simulink library "aausat3_lib"  (Simulink 8.3)
settings: Solver=ode45  StartTime=0.0  StopTime=10.0  RelTol=1e-3
undefined symbols (not defined in the file or in its folder): A_wire_mt, albedo_wrapper, alpha_0_mt, bias_gyro, bias_mag, bias_sun, Cd, coil_dim, Dim, f_sample, G, heading_gyro, heading_mag, M_earth, M_moon, M_sun, magnitude, n_mt, noise_gyro, noise_mag, noise_sun, nr_sample_sun, otoquest, otoquest_with_pro, q_method, qmethod, redfac, refldata, s_freq_gyro, s_freq_mag, s_freq_sun, sigma_0_mt, solar_absorb_coeff, solar_m_flux, SVD_method, T_0_mt, theta_e, tilt_gyro, tilt_mag, Ts
undefined symbols (not defined in the file): Actuator_Duty_Cycle_coil, Actuator_Frequency_coil, Dimensions_coil, mean_refl, Number_of_Windings_coil, rho, sim_par, svd_weigth, Wire_Cross_Sectional_Area_coil, Wire_Resistivity_Base_Temperature_coil, Wire_Resistivity_coil, Wire_Resistivity_Temperature_Coefficient_coil
libraries: aausat3_lib x118, simulink_extras x3
(part 4 of 4)

== system aausat3_lib/On-board Software/Orbit and Magnetic field models/initial time ==
  Initial time in (JD) : Inport
  TLE : Inport  Port=2
  Demux : Demux  Outputs=12
  Mux1 : Mux  Inputs=12
  Switch : Switch  Criteria=u2 > Threshold
  "TLE -> JD converter SW" : aausat3_lib/Other Model Utilities/TLE -> JD converter  SystemSampleTime=-1
  Terminator : Terminator
  Initial time out (JD) : Outport
  wires:
  Mux1/1 -> Terminator/1
  Switch/1 -> Initial time out (JD)/1
  Initial time in (JD)/1 -> Switch/1, Switch/2
  TLE/1 -> Demux/1
  Demux/2 -> Mux1/2
  Demux/3 -> Mux1/3
  Demux/4 -> Mux1/4
  Demux/5 -> Mux1/5
  Demux/6 -> Mux1/6
  Demux/7 -> Mux1/7
  Demux/8 -> Mux1/8
  Demux/9 -> Mux1/9
  Demux/10 -> Mux1/10
  Demux/11 -> Mux1/11
  Demux/12 -> Mux1/12
  Demux/1 -> "TLE -> JD converter SW"/1
  "TLE -> JD converter SW"/1 -> Switch/3, Mux1/1

== system aausat3_lib/Orbit and Ephemeris/(IGRF) Magnetic field/Magnetic field model ==
  R_sc(E) : Inport
  S-Function : S-Function  FunctionName=igrfS  Parameters=2009,13  EnableBusSupport=off
  B(E) : Outport
  wires:
  R_sc(E)/1 -> S-Function/1
  S-Function/1 -> B(E)/1

== system aausat3_lib/Orbit and Ephemeris/Albedo/Earth Albedo Model ==
  r_sat_ecef : Inport  SampleTime=Ts
  r_sun_ecef : Inport  Port=2  SampleTime=Ts
  AlbedoFcn : MATLABFcn  MATLABFcn=albedo_wrapper(u(1:3),u(4:6),refldata,redfac)  OutputDimensions=[sy sx]  OutputSignalType=real  Output1D=off
  Mux : Mux  Inputs=2
  Zero-Order Hold1 : ZeroOrderHold  SampleTime=Ts
  Zero-Order Hold2 : ZeroOrderHold  SampleTime=Ts
  a : Outport
  wires:
  r_sat_ecef/1 -> Zero-Order Hold2/1
  AlbedoFcn/1 -> a/1
  r_sun_ecef/1 -> Zero-Order Hold1/1
  Zero-Order Hold2/1 -> Mux/1
  Zero-Order Hold1/1 -> Mux/2
  Mux/1 -> AlbedoFcn/1

== system aausat3_lib/Orbit and Ephemeris/Ephemeris/Moon Position ==
  t(JD)1 : Inport
  MATLAB Function : MATLAB Function  TreatAsAtomicUnit=on
  R_m(I) : Outport
  wires:
  MATLAB Function/1(y) -> R_m(I)/1
  t(JD)1/1 -> MATLAB Function/1(u)

== system aausat3_lib/Orbit and Ephemeris/Ephemeris/Sun Position ==
  t(JD) : Inport
  MATLAB Function : MATLAB Function  TreatAsAtomicUnit=on
  R_s(I) : Outport
  wires:
  MATLAB Function/1(y) -> R_s(I)/1
  t(JD)/1 -> MATLAB Function/1(u)

== system aausat3_lib/Orbit and Ephemeris/Orbit and Magnetic field models/initial time ==
  Initial time in (JD) : Inport
  TLE : Inport  Port=2
  Demux : Demux  Outputs=12
  Mux1 : Mux  Inputs=12
  Switch : Switch  Criteria=u2 > Threshold
  "TLE -> JD converter" : aausat3_lib/Other Model Utilities/TLE -> JD converter
  Terminator : Terminator
  Initial time out (JD) : Outport
  wires:
  "TLE -> JD converter"/1 -> Mux1/1, Switch/3
  Demux/1 -> "TLE -> JD converter"/1
  Demux/12 -> Mux1/12
  Demux/11 -> Mux1/11
  Demux/10 -> Mux1/10
  Demux/9 -> Mux1/9
  Demux/8 -> Mux1/8
  Demux/7 -> Mux1/7
  Demux/6 -> Mux1/6
  Demux/5 -> Mux1/5
  Demux/4 -> Mux1/4
  Demux/3 -> Mux1/3
  Demux/2 -> Mux1/2
  TLE/1 -> Demux/1
  Initial time in (JD)/1 -> Switch/2, Switch/1
  Switch/1 -> Initial time out (JD)/1
  Mux1/1 -> Terminator/1

== system aausat3_lib/Other Model Utilities/Exposed area/Projection Matrix1 ==
  n-vector : Inport
  Add : Sum  Inputs=+++
  Demux : Demux  Outputs=3
  Gain{1..6} (6 alike) : Gain  Gain=-1
  Math Funcion : Math  Operator=square  SaturateOnIntegerOverflow=on
  Math Function : Math  Operator=reciprocal  SaturateOnIntegerOverflow=on
  Math Function1 : Math  Operator=square  SaturateOnIntegerOverflow=on
  Math Function2 : Math  Operator=square  SaturateOnIntegerOverflow=on
  Mux : Mux  Inputs=9
  Product1 : Product  RndMeth=Zero
  Product2 : Product  RndMeth=Zero
  Product3 : Product  RndMeth=Zero
  Prouct : Product  RndMeth=Zero
  Reshape : Reshape  OutputDimensionality=Customize  OutputDimensions=[3,3]
  Sum : Sum  Inputs=|++
  Sum1 : Sum  Inputs=+|+
  Sum2 : Sum  Inputs=++|
  P matrix : Outport
  wires:
  Prouct/1 -> P matrix/1
  Reshape/1 -> Prouct/2
  Add/1 -> Math Function/1
  Math Function/1 -> Prouct/1
  n-vector/1 -> Demux/1
  Mux/1 -> Reshape/1
  Math Function1/1 -> Add/2, Sum/1, Sum2/2
  Math Function2/1 -> Add/3, Sum/2, Sum1/2
  Math Funcion/1 -> Add/1, Sum2/1, Sum1/1
  Sum1/1 -> Mux/5
  Sum2/1 -> Mux/9
  Sum/1 -> Mux/1
  Product3/1 -> Gain6/1, Gain4/1
  Product2/1 -> Gain5/1, Gain2/1
  Product1/1 -> Gain3/1, Gain1/1
  Gain6/1 -> Mux/8
  Gain5/1 -> Mux/7
  Gain4/1 -> Mux/6
  Gain3/1 -> Mux/4
  Gain2/1 -> Mux/3
  Gain1/1 -> Mux/2
  Demux/3 -> Product3/2, Math Function2/1, Product2/2
  Demux/2 -> Product3/1, Product1/2, Math Function1/1
  Demux/1 -> Product2/1, Product1/1, Math Funcion/1

== system aausat3_lib/Other Model Utilities/Geocentric to  Geodetic Latitude/alt ==
  l_point : Inport
  delta_lambda : Inport  Port=2
  Product : Product  RndMeth=Zero
  Trigonometric Function1 : Trigonometry  Operator=cos
  alt : Outport
  wires:
  Trigonometric Function1/1 -> Product/2
  l_point/1 -> Product/1
  Product/1 -> alt/1
  delta_lambda/1 -> Trigonometric Function1/1

== system aausat3_lib/Other Model Utilities/Geocentric to  Geodetic Latitude/delt_mu ==
  l_point : Inport
  alt : Inport  Port=2
  delta_lambda : Inport  Port=3
  rho_alpha : Inport  Port=4
  Product : Product  RndMeth=Zero
  Sum1 : Sum  Inputs=|++
  Trigonometric Function1 : Trigonometry  Operator=atan2
  Trigonometric Function2 : Trigonometry
  delt_mu : Outport
  wires:
  Product/1 -> Trigonometric Function1/1
  l_point/1 -> Product/1
  delta_lambda/1 -> Trigonometric Function2/1
  alt/1 -> Sum1/1
  Sum1/1 -> Trigonometric Function1/2
  rho_alpha/1 -> Sum1/2
  Trigonometric Function1/1 -> delt_mu/1
  Trigonometric Function2/1 -> Product/2

== system aausat3_lib/Other Model Utilities/Geocentric to  Geodetic Latitude/delta_lambda ==
  mu_alpha : Inport
  lambda : Inport  Port=2
  Sum1 : Sum  Inputs=|+-
  delta_lambda : Outport
  wires:
  lambda/1 -> Sum1/2
  mu_alpha/1 -> Sum1/1
  Sum1/1 -> delta_lambda/1

== system aausat3_lib/Other Model Utilities/Geocentric to  Geodetic Latitude/denom ==
  mu_alpha : Inport
  eps : Inport  Port=2
  Constant : Constant
  Math Function : Math  Operator=sqrt  SaturateOnIntegerOverflow=on
  Product1 : Product  Inputs=4  RndMeth=Zero
  Sum1 : Sum  Inputs=|+-
  Trigonometric Function1 : Trigonometry
  denom : Outport
  wires:
  Math Function/1 -> denom/1
  Sum1/1 -> Math Function/1
  Constant/1 -> Sum1/1
  Product1/1 -> Sum1/2
  eps/1 -> Product1/2, Product1/1
  Trigonometric Function1/1 -> Product1/4, Product1/3
  mu_alpha/1 -> Trigonometric Function1/1

== system aausat3_lib/Other Model Utilities/Geocentric to  Geodetic Latitude/e ==
  Constant : Constant  Value=F
  Sum : Sum  Inputs=-+
  f : Constant
  e : Outport
  wires:
  Sum/1 -> e/1
  Constant/1 -> Sum/1
  f/1 -> Sum/2

== system aausat3_lib/Other Model Utilities/Geocentric to  Geodetic Latitude/e^4 ==
  e : Inport
  Constant : Constant
  Math Function : Math  Operator=sqrt  SaturateOnIntegerOverflow=on
  Product1 : Product  RndMeth=Zero
  Sum1 : Sum  Inputs=|+-
  eps : Outport
  wires:
  e/1 -> Product1/1, Product1/2
  Product1/1 -> Sum1/2
  Constant/1 -> Sum1/1
  Sum1/1 -> Math Function/1
  Math Function/1 -> eps/1

== system aausat3_lib/Other Model Utilities/Geocentric to  Geodetic Latitude/l_point ==
  dist to body : Inport
  r_alpha : Inport  Port=2
  Sum1 : Sum  Inputs=|+-
  l_point : Outport
  wires:
  Sum1/1 -> l_point/1
  dist to body/1 -> Sum1/1
  r_alpha/1 -> Sum1/2

== system aausat3_lib/Other Model Utilities/Geocentric to  Geodetic Latitude/mu_alpha ==
  R^2 : Inport
  x_alpha : Inport  Port=2
  e : Inport  Port=3
  lambda : Inport  Port=4
  Math Function1 : Math  Operator=sqrt  SaturateOnIntegerOverflow=on
  Product1 : Product  RndMeth=Zero
  Product2 : Product  RndMeth=Zero
  Product3 : Product  RndMeth=Zero
  Sign : Signum
  Sum1 : Sum  Inputs=+-|
  Trigonometric Function1 : Trigonometry  Operator=atan2
  mu_alpha : Outport
  wires:
  x_alpha/1 -> Product3/1, Product2/1, Product2/2  "x_alpha"
  Product2/1 -> Sum1/2
  Sum1/1 -> Math Function1/1
  Math Function1/1 -> Trigonometric Function1/1
  Product3/1 -> Trigonometric Function1/2
  e/1 -> Product3/2
  R^2/1 -> Sum1/1
  Product1/1 -> mu_alpha/1  "mu_alpha"
  lambda/1 -> Sign/1
  Trigonometric Function1/1 -> Product1/1  "mu_alpha"
  Sign/1 -> Product1/2

== system aausat3_lib/Other Model Utilities/Geocentric to  Geodetic Latitude/r_alpha ==
  lambda : Inport
  x_alpha : Inport  Port=2
  Product : Product  Inputs=*/  RndMeth=Zero
  Trigonometric Function1 : Trigonometry  Operator=cos
  r_alpha : Outport
  wires:
  Trigonometric Function1/1 -> Product/2
  lambda/1 -> Trigonometric Function1/1
  x_alpha/1 -> Product/1
  Product/1 -> r_alpha/1

== system aausat3_lib/Other Model Utilities/Geocentric to  Geodetic Latitude/rho_alpha ==
  R : Inport
  denom : Inport  Port=2
  eps : Inport  Port=3
  Constant1 : Constant
  Product1 : Product  Inputs=**/  RndMeth=Zero
  Product2 : Product  Inputs=**  RndMeth=Zero
  Product3 : Product  Inputs=3  RndMeth=Zero
  Sum1 : Sum  Inputs=|+-
  rho_alpha : Outport
  wires:
  denom/1 -> Product3/1, Product3/2, Product3/3
  Constant1/1 -> Sum1/1
  Sum1/1 -> Product1/2
  R/1 -> Product1/1
  eps/1 -> Product2/1, Product2/2
  Product1/1 -> rho_alpha/1
  Product2/1 -> Sum1/2
  Product3/1 -> Product1/3

== system aausat3_lib/Other Model Utilities/Geocentric to  Geodetic Latitude/square e ==
  e : Inport
  Product1 : Product  Inputs=**  RndMeth=Zero
  e^2 : Outport
  wires:
  Product1/1 -> e^2/1
  e/1 -> Product1/2, Product1/1

== system aausat3_lib/Other Model Utilities/Geocentric to  Geodetic Latitude/square e1 ==
  R : Inport
  Product1 : Product  Inputs=**  RndMeth=Zero
  R^2 : Outport
  wires:
  R/1 -> Product1/1, Product1/2
  Product1/1 -> R^2/1

== system aausat3_lib/Other Model Utilities/Geocentric to  Geodetic Latitude/x_alpha ==
  R : Inport
  t_lat : Inport  Port=2
  e : Inport  Port=3
  e^2 : Inport  Port=4
  Math Function : Math  Operator=sqrt  SaturateOnIntegerOverflow=on
  Product : Product  RndMeth=Zero
  Product1 : Product  Inputs=*/*  RndMeth=Zero
  Sum : Sum  Inputs=|++
  x_alpha : Outport
  wires:
  t_lat/1 -> Product/1, Product/2  "t_lat"
  Product/1 -> Sum/1
  Sum/1 -> Math Function/1
  Math Function/1 -> Product1/2
  R/1 -> Product1/1
  e/1 -> Product1/3
  Product1/1 -> x_alpha/1  "x_alpha"
  e^2/1 -> Sum/2

== system aausat3_lib/Other Model Utilities/Geodetic to  Geocentric Latitude/Radius at Geocentric Latitude ==
  lambda_s : Inport
  Constant : Constant
  Math Function : Math  Operator=sqrt  SaturateOnIntegerOverflow=on
  Product1 : Product  Inputs=*/  RndMeth=Zero
  Product2 : Product  Inputs=3  RndMeth=Zero
  Product3 : Product  Inputs=**/  RndMeth=Zero
  Product4 : Product  RndMeth=Zero
  Re : Constant  Value=R
  Sum : Sum  Inputs=+-
  Sum1 : Sum  Inputs=-+|
  Sum2 : Sum  Inputs=++|
  Trigonometric Function : Trigonometry
  deg->rad : Gain  Gain=pi/180
  f : Constant  Value=F
  r_s : Outport
  wires:
  Product4/1 -> Product1/2
  lambda_s/1 -> deg->rad/1
  Constant/1 -> Product1/1, Sum/1, Sum1/1, Sum2/1
  f/1 -> Sum/2
  Sum/1 -> Product4/1, Product4/2
  Product1/1 -> Sum1/2
  Sum1/1 -> Product2/3
  Trigonometric Function/1 -> Product2/1, Product2/2
  Product2/1 -> Sum2/2
  Sum2/1 -> Product3/3
  Re/1 -> Product3/2, Product3/1
  Product3/1 -> Math Function/1
  Math Function/1 -> r_s/1
  deg->rad/1 -> Trigonometric Function/1

== system aausat3_lib/Other Model Utilities/Store data/enable ==
  In : Inport
  Constant : Constant  Value=enable_signal
  Ground : Ground
  Switch : Switch  Threshold=1
  Out : Outport
  wires:
  Constant/1 -> Switch/2
  Ground/1 -> Switch/3
  In/1 -> Switch/1
  Switch/1 -> Out/1

== system aausat3_lib/Other Model Utilities/Store data/enable1 ==
  In : Inport
  Constant : Constant  Value=enable_signal
  Ground : Ground
  Switch : Switch  Threshold=1
  Out : Outport
  wires:
  Constant/1 -> Switch/2
  Ground/1 -> Switch/3
  In/1 -> Switch/1
  Switch/1 -> Out/1

== system aausat3_lib/Other Model Utilities/Store data/enable10 ==
  In : Inport
  Constant : Constant  Value=enable_signal
  Ground : Ground
  Switch : Switch  Threshold=1
  Out : Outport
  wires:
  Constant/1 -> Switch/2
  Ground/1 -> Switch/3
  In/1 -> Switch/1
  Switch/1 -> Out/1

== system aausat3_lib/Other Model Utilities/Store data/enable11 ==
  In : Inport
  Constant : Constant  Value=enable_signal
  Ground : Ground
  Switch : Switch  Threshold=1
  Out : Outport
  wires:
  Constant/1 -> Switch/2
  Ground/1 -> Switch/3
  In/1 -> Switch/1
  Switch/1 -> Out/1

== system aausat3_lib/Other Model Utilities/Store data/enable12 ==
  In : Inport
  Constant : Constant  Value=enable_signal
  Ground : Ground
  Switch : Switch  Threshold=1
  Out : Outport
  wires:
  Constant/1 -> Switch/2
  Ground/1 -> Switch/3
  In/1 -> Switch/1
  Switch/1 -> Out/1

== system aausat3_lib/Other Model Utilities/Store data/enable13 ==
  In : Inport
  Constant : Constant  Value=enable_signal
  Ground : Ground
  Switch : Switch  Threshold=1
  Out : Outport
  wires:
  Constant/1 -> Switch/2
  Ground/1 -> Switch/3
  In/1 -> Switch/1
  Switch/1 -> Out/1

== system aausat3_lib/Other Model Utilities/Store data/enable14 ==
  In : Inport
  Constant : Constant  Value=enable_signal
  Ground : Ground
  Switch : Switch  Threshold=1
  Out : Outport
  wires:
  Constant/1 -> Switch/2
  Ground/1 -> Switch/3
  In/1 -> Switch/1
  Switch/1 -> Out/1

== system aausat3_lib/Other Model Utilities/Store data/enable15 ==
  In : Inport
  Constant : Constant  Value=enable_signal
  Ground : Ground
  Switch : Switch  Threshold=1
  Out : Outport
  wires:
  Constant/1 -> Switch/2
  Ground/1 -> Switch/3
  In/1 -> Switch/1
  Switch/1 -> Out/1

== system aausat3_lib/Other Model Utilities/Store data/enable16 ==
  In : Inport
  Constant : Constant  Value=enable_signal
  Ground : Ground
  Switch : Switch  Threshold=1
  Out : Outport
  wires:
  Constant/1 -> Switch/2
  Ground/1 -> Switch/3
  In/1 -> Switch/1
  Switch/1 -> Out/1

== system aausat3_lib/Other Model Utilities/Store data/enable17 ==
  In : Inport
  Constant : Constant  Value=enable_signal
  Ground : Ground
  Switch : Switch  Threshold=1
  Out : Outport
  wires:
  Constant/1 -> Switch/2
  Ground/1 -> Switch/3
  In/1 -> Switch/1
  Switch/1 -> Out/1

== system aausat3_lib/Other Model Utilities/Store data/enable18 ==
  In : Inport
  Constant : Constant  Value=enable_signal
  Ground : Ground
  Switch : Switch  Threshold=1
  Out : Outport
  wires:
  Constant/1 -> Switch/2
  Ground/1 -> Switch/3
  In/1 -> Switch/1
  Switch/1 -> Out/1

== system aausat3_lib/Other Model Utilities/Store data/enable19 ==
  In : Inport
  Constant : Constant  Value=enable_signal
  Ground : Ground
  Switch : Switch  Threshold=1
  Out : Outport
  wires:
  Constant/1 -> Switch/2
  Ground/1 -> Switch/3
  In/1 -> Switch/1
  Switch/1 -> Out/1

== system aausat3_lib/Other Model Utilities/Store data/enable2 ==
  In : Inport
  Constant : Constant  Value=enable_signal
  Ground : Ground
  Switch : Switch  Threshold=1
  Out : Outport
  wires:
  Constant/1 -> Switch/2
  Ground/1 -> Switch/3
  In/1 -> Switch/1
  Switch/1 -> Out/1

== system aausat3_lib/Other Model Utilities/Store data/enable21 ==
  In : Inport
  Constant : Constant  Value=enable_signal
  Ground : Ground
  Switch : Switch  Threshold=1
  Out : Outport
  wires:
  Constant/1 -> Switch/2
  Ground/1 -> Switch/3
  In/1 -> Switch/1
  Switch/1 -> Out/1

== system aausat3_lib/Other Model Utilities/Store data/enable22 ==
  In : Inport
  Constant : Constant  Value=enable_signal
  Ground : Ground
  Switch : Switch  Threshold=1
  Out : Outport
  wires:
  Constant/1 -> Switch/2
  Ground/1 -> Switch/3
  In/1 -> Switch/1
  Switch/1 -> Out/1

== system aausat3_lib/Other Model Utilities/Store data/enable23 ==
  In : Inport
  Constant : Constant  Value=enable_signal
  Ground : Ground
  Switch : Switch  Threshold=1
  Out : Outport
  wires:
  Constant/1 -> Switch/2
  Ground/1 -> Switch/3
  In/1 -> Switch/1
  Switch/1 -> Out/1

== system aausat3_lib/Other Model Utilities/Store data/enable24 ==
  In : Inport
  Constant : Constant  Value=enable_signal
  Ground : Ground
  Switch : Switch  Threshold=1
  Out : Outport
  wires:
  Constant/1 -> Switch/2
  Ground/1 -> Switch/3
  In/1 -> Switch/1
  Switch/1 -> Out/1

== system aausat3_lib/Other Model Utilities/Store data/enable25 ==
  In : Inport
  Constant : Constant  Value=enable_signal
  Ground : Ground
  Switch : Switch  Threshold=1
  Out : Outport
  wires:
  Constant/1 -> Switch/2
  Ground/1 -> Switch/3
  In/1 -> Switch/1
  Switch/1 -> Out/1

== system aausat3_lib/Other Model Utilities/Store data/enable26 ==
  In : Inport
  Constant : Constant  Value=enable_signal
  Ground : Ground
  Switch : Switch  Threshold=1
  Out : Outport
  wires:
  Constant/1 -> Switch/2
  Ground/1 -> Switch/3
  In/1 -> Switch/1
  Switch/1 -> Out/1

== system aausat3_lib/Other Model Utilities/Store data/enable27 ==
  In : Inport
  Constant : Constant  Value=enable_signal
  Ground : Ground
  Switch : Switch  Threshold=1
  Out : Outport
  wires:
  Constant/1 -> Switch/2
  Ground/1 -> Switch/3
  In/1 -> Switch/1
  Switch/1 -> Out/1

== system aausat3_lib/Other Model Utilities/Store data/enable28 ==
  In : Inport
  Constant : Constant  Value=enable_signal
  Ground : Ground
  Switch : Switch  Threshold=1
  Out : Outport
  wires:
  Constant/1 -> Switch/2
  Ground/1 -> Switch/3
  In/1 -> Switch/1
  Switch/1 -> Out/1

== system aausat3_lib/Other Model Utilities/Store data/enable29 ==
  In : Inport
  Constant : Constant  Value=enable_signal
  Ground : Ground
  Switch : Switch  Threshold=1
  Out : Outport
  wires:
  Constant/1 -> Switch/2
  Ground/1 -> Switch/3
  In/1 -> Switch/1
  Switch/1 -> Out/1

== system aausat3_lib/Other Model Utilities/Store data/enable3 ==
  In : Inport
  Constant : Constant  Value=enable_signal
  Ground : Ground
  Switch : Switch  Threshold=1
  Out : Outport
  wires:
  Constant/1 -> Switch/2
  Ground/1 -> Switch/3
  In/1 -> Switch/1
  Switch/1 -> Out/1

== system aausat3_lib/Other Model Utilities/Store data/enable4 ==
  In : Inport
  Constant : Constant  Value=enable_signal
  Ground : Ground
  Switch : Switch  Threshold=1
  Out : Outport
  wires:
  Constant/1 -> Switch/2
  Ground/1 -> Switch/3
  In/1 -> Switch/1
  Switch/1 -> Out/1

== system aausat3_lib/Other Model Utilities/Store data/enable5 ==
  In : Inport
  Constant : Constant  Value=enable_signal
  Ground : Ground
  Switch : Switch  Threshold=1
  Out : Outport
  wires:
  Constant/1 -> Switch/2
  Ground/1 -> Switch/3
  In/1 -> Switch/1
  Switch/1 -> Out/1

== system aausat3_lib/Other Model Utilities/Store data/enable6 ==
  In : Inport
  Constant : Constant  Value=enable_signal
  Ground : Ground
  Switch : Switch  Threshold=1
  Out : Outport
  wires:
  Constant/1 -> Switch/2
  Ground/1 -> Switch/3
  In/1 -> Switch/1
  Switch/1 -> Out/1

== system aausat3_lib/Other Model Utilities/Store data/enable7 ==
  In : Inport
  Constant : Constant  Value=enable_signal
  Ground : Ground
  Switch : Switch  Threshold=1
  Out : Outport
  wires:
  Constant/1 -> Switch/2
  Ground/1 -> Switch/3
  In/1 -> Switch/1
  Switch/1 -> Out/1

== system aausat3_lib/Other Model Utilities/Store data/enable8 ==
  In : Inport
  Constant : Constant  Value=enable_signal
  Ground : Ground
  Switch : Switch  Threshold=1
  Out : Outport
  wires:
  Constant/1 -> Switch/2
  Ground/1 -> Switch/3
  In/1 -> Switch/1
  Switch/1 -> Out/1

== system aausat3_lib/Other Model Utilities/Store data/enable9 ==
  In : Inport
  Constant : Constant  Value=enable_signal
  Ground : Ground
  Switch : Switch  Threshold=1
  Out : Outport
  wires:
  Constant/1 -> Switch/2
  Ground/1 -> Switch/3
  In/1 -> Switch/1
  Switch/1 -> Out/1

== system aausat3_lib/Sensor Emulation/Magnetometers/Vector rotation by q ==
  q : Inport
  V : Inport  Port=2
  Constant : Constant  Value=0
  Demux : Demux  Outputs=3
  Demux1 : Demux
  Mux : Mux
  Mux1 : Mux  Inputs=3
  Quaternion inverter : Subsystem
  Quaternion mulitiplication : S-Function  FunctionName=qmul  EnableBusSupport=off
  Quaternion mulitiplication1 : S-Function  FunctionName=qmul  EnableBusSupport=off
  Terminator : Terminator
  q'Vq : Outport
  wires:
  Mux1/1 -> q'Vq/1
  Demux1/4 -> Terminator/1
  Demux1/3 -> Mux1/3
  Demux1/2 -> Mux1/2
  Demux1/1 -> Mux1/1
  Quaternion mulitiplication1/1 -> Demux1/1
  Quaternion mulitiplication/1 -> Quaternion mulitiplication1/1
  Mux/1 -> Quaternion mulitiplication/2
  Constant/1 -> Mux/4
  Demux/3 -> Mux/3
  Demux/2 -> Mux/2
  Demux/1 -> Mux/1
  V/1 -> Demux/1
  Quaternion inverter/1(q^-1) -> Quaternion mulitiplication/1
  q/1 -> Quaternion mulitiplication1/2, Quaternion inverter/1(q)

== system aausat3_lib/Sensor Emulation/Sun sensors/Cartesian to Spherical ==
  x : Inport  PortDimensions=1
  y : Inport  Port=2  PortDimensions=1
  z : Inport  Port=3  PortDimensions=1
  Mux : Mux  Inputs=2
  Mux1 : Mux  Inputs=2
  calc phi : Fcn  Expr=atan2(u[1],u[2])
  calc r : Fcn  Expr=hypot(u[1],u[2])
  calc theta : Fcn  Expr=atan2(u[2],u[1])
  temp : Fcn  Expr=hypot(u[1],u[2])
  "r " : Outport  InitialOutput=0
  theta : Outport  Port=2  InitialOutput=0
  phi : Outport  Port=3  InitialOutput=0
  wires:
  calc theta/1 -> theta/1
  calc phi/1 -> phi/1
  y/1 -> Mux/2
  x/1 -> Mux/1
  temp/1 -> Mux1/1
  z/1 -> Mux1/2
  calc r/1 -> "r "/1
  Mux/1 -> calc theta/1, temp/1
  Mux1/1 -> calc phi/1, calc r/1

== system aausat3_lib/Sensor Emulation/Sun sensors/Spherical to Cartesian ==
  r : Inport  PortDimensions=1
  theta : Inport  Port=2  PortDimensions=1
  phi : Inport  Port=3  PortDimensions=1
  Mux : Mux  Inputs=2
  Mux1 : Mux  Inputs=2
  temp : Fcn  Expr=u[1]*sin(u[2])
  x : Fcn  Expr=u[1]*cos(u[2])
  y : Fcn  Expr=u[1]*sin(u[2])
  z : Fcn  Expr=u[1]*cos(u[2])
  X : Outport  InitialOutput=0
  Y : Outport  Port=2  InitialOutput=0
  Z : Outport  Port=3  InitialOutput=0
  wires:
  z/1 -> Z/1
  y/1 -> Y/1
  x/1 -> X/1
  temp/1 -> Mux1/1
  r/1 -> Mux/1
  phi/1 -> Mux/2
  theta/1 -> Mux1/2
  Mux1/1 -> y/1, x/1
  Mux/1 -> z/1, temp/1

== system aausat3_lib/Sensor Emulation/Sun sensors/Vector rotation by q ==
  q : Inport
  V : Inport  Port=2
  Constant : Constant  Value=0
  Demux : Demux  Outputs=3
  Demux1 : Demux
  Mux : Mux
  Mux1 : Mux  Inputs=3
  Quaternion inverter : Subsystem
  Quaternion mulitiplication : S-Function  FunctionName=qmul  EnableBusSupport=off
  Quaternion mulitiplication1 : S-Function  FunctionName=qmul  EnableBusSupport=off
  Terminator : Terminator
  q'Vq : Outport
  wires:
  Mux1/1 -> q'Vq/1
  Demux1/4 -> Terminator/1
  Demux1/3 -> Mux1/3
  Demux1/2 -> Mux1/2
  Demux1/1 -> Mux1/1
  Quaternion mulitiplication1/1 -> Demux1/1
  Quaternion mulitiplication/1 -> Quaternion mulitiplication1/1
  Mux/1 -> Quaternion mulitiplication/2
  Constant/1 -> Mux/4
  Demux/3 -> Mux/3
  Demux/2 -> Mux/2
  Demux/1 -> Mux/1
  V/1 -> Demux/1
  Quaternion inverter/1(q^-1) -> Quaternion mulitiplication/1
  q/1 -> Quaternion mulitiplication1/2, Quaternion inverter/1(q)

== system aausat3_lib/Actuator Emulation/Permanent Magnet/Vector rotation by q/Quaternion inverter ==
  q : Inport
  Demux : Demux
  Demux1 : Demux  Outputs=3
  Gain : Gain  Gain=-1  SaturateOnIntegerOverflow=on  OutDataTypeStr=Inherit: Same as input  ParamDataTypeStr=Inherit: Same as input
  Mux : Mux
  Mux1 : Mux  Inputs=3
  q^-1 : Outport
  wires:
  Gain/1 -> Demux1/1
  Demux1/3 -> Mux/3
  Demux1/2 -> Mux/2
  Demux1/1 -> Mux/1
  Mux1/1 -> Gain/1
  Demux/3 -> Mux1/3
  Demux/2 -> Mux1/2
  Demux/1 -> Mux1/1
  Demux/4 -> Mux/4
  Mux/1 -> q^-1/1
  q/1 -> Demux/1

== system aausat3_lib/Disturbances/Atmospheric/Density7/Exponent n Eq: [(1/22.5)*i]+2 ==
  i : Inport
  Add : Sum
  Product : Product  RndMeth=Zero
  a : Constant  Value=1/22.5
  b : Constant  Value=2
  n : Outport
  wires:
  Add/1 -> n/1
  i/1 -> Product/1
  b/1 -> Add/2
  Product/1 -> Add/1
  a/1 -> Product/2

== system aausat3_lib/Disturbances/Atmospheric/Density7/Subsystem ==
  JD : Inport
  30 deg Lag Angle in Longitude : Constant  Value=30*(pi/180)
  Add1 : Sum
  Add2 : Sum
  Clock : Clock
  Constant3 : Constant  Value=86400
  Display : Display
  Display1 : Display
  Display2 : Display
  Divide2 : Product  Inputs=*/
  Mux : Mux  Inputs=3
  Product : Product  RndMeth=Zero
  Product1 : Product  RndMeth=Zero
  R.Ascen & Declination in rads : MATLAB Function  TreatAsAtomicUnit=on
  Trigonometric Function : Trigonometry
  Trigonometric Function1 : Trigonometry  Operator=cos
  Trigonometric Function2 : Trigonometry
  Trigonometric Function3 : Trigonometry  Operator=cos
  e-sun : Outport
  wires:
  Mux/1 -> Display/1, e-sun/1
  Trigonometric Function2/1 -> Mux/3
  Product1/1 -> Mux/2
  Product/1 -> Mux/1
  Trigonometric Function/1 -> Product1/1
  Trigonometric Function3/1 -> Product1/2, Product/2
  Trigonometric Function1/1 -> Product/1
  R.Ascen & Declination in rads/2(decl) -> Trigonometric Function2/1, Trigonometric Function3/1, Display1/1
  Add2/1 -> Trigonometric Function1/1, Trigonometric Function/1
  R.Ascen & Declination in rads/1(rtasc) -> Display2/1, Add2/2
  30 deg Lag Angle in Longitude/1 -> Add2/1
  Add1/1 -> R.Ascen & Declination in rads/1(jd)
  JD/1 -> Add1/1
  Divide2/1 -> Add1/2
  Constant3/1 -> Divide2/2
  Clock/1 -> Divide2/1

== system aausat3_lib/Disturbances/Atmospheric/Density7/Unit Vector ==
  Vector : Inport
  Divide1 : Product  Inputs=*/
  Vector Mag : Subsystem
  Unit Vector : Outport
  wires:
  Divide1/1 -> Unit Vector/1
  Vector/1 -> Vector Mag/1(Vector), Divide1/1
  Vector Mag/1(Magnitude) -> Divide1/2

== system aausat3_lib/Math Utilities/Quaternion operations/Rotation from q1 to q2/Quaternion inverter ==
  q : Inport
  Demux : Demux
  Demux1 : Demux  Outputs=3
  Gain : Gain  Gain=-1  SaturateOnIntegerOverflow=on  OutDataTypeStr=Inherit: Same as input  ParamDataTypeStr=Inherit: Same as input
  Mux : Mux
  Mux1 : Mux  Inputs=3
  q^-1 : Outport
  wires:
  Gain/1 -> Demux1/1
  Demux1/3 -> Mux/3
  Demux1/2 -> Mux/2
  Demux1/1 -> Mux/1
  Mux1/1 -> Gain/1
  Demux/3 -> Mux1/3
  Demux/2 -> Mux1/2
  Demux/1 -> Mux1/1
  Demux/4 -> Mux/4
  Mux/1 -> q^-1/1
  q/1 -> Demux/1

== system aausat3_lib/Math Utilities/Quaternion operations/Vector rotation by q/Quaternion inverter ==
  q : Inport
  Demux : Demux
  Demux1 : Demux  Outputs=3
  Gain : Gain  Gain=-1  SaturateOnIntegerOverflow=on  OutDataTypeStr=Inherit: Same as input  ParamDataTypeStr=Inherit: Same as input
  Mux : Mux
  Mux1 : Mux  Inputs=3
  q^-1 : Outport
  wires:
  q/1 -> Demux/1
  Mux/1 -> q^-1/1
  Demux/4 -> Mux/4
  Demux/1 -> Mux1/1
  Demux/2 -> Mux1/2
  Demux/3 -> Mux1/3
  Mux1/1 -> Gain/1
  Demux1/1 -> Mux/1
  Demux1/2 -> Mux/2
  Demux1/3 -> Mux/3
  Gain/1 -> Demux1/1

== system aausat3_lib/Math Utilities/Quaternion operations/quaternion composition/to unit vector ==
  "v  " : Inport
  Constant : Constant
  Dot Product : DotProduct  InputSameDT=on  OutDataTypeStr=Inherit: Inherit via internal rule
  Math Function : Math  Operator=reciprocal  SaturateOnIntegerOverflow=on
  Product : Product  SaturateOnIntegerOverflow=on  OutDataTypeStr=Inherit: Same as first input
  Switch : Switch  Criteria=u2 ~= 0  SaturateOnIntegerOverflow=on
  sqrt : Math  Operator=sqrt  SaturateOnIntegerOverflow=on
  v_hat : Outport
  wires:
  Dot Product/1 -> sqrt/1
  Product/1 -> v_hat/1
  Math Function/1 -> Product/2
  "v  "/1 -> Dot Product/2, Dot Product/1, Product/1
  Switch/1 -> Math Function/1
  sqrt/1 -> Switch/2, Switch/1
  Constant/1 -> Switch/3

== system aausat3_lib/Math Utilities/Quaternion operations/quaternion decomposition/to unit vector ==
  "v  " : Inport
  Constant : Constant
  Dot Product : DotProduct  InputSameDT=on  OutDataTypeStr=Inherit: Inherit via internal rule
  Math Function : Math  Operator=reciprocal  SaturateOnIntegerOverflow=on
  Product : Product  SaturateOnIntegerOverflow=on  OutDataTypeStr=Inherit: Same as first input
  Switch : Switch  Criteria=u2 ~= 0  SaturateOnIntegerOverflow=on
  sqrt : Math  Operator=sqrt  SaturateOnIntegerOverflow=on
  v_hat : Outport
  wires:
  Dot Product/1 -> sqrt/1
  Product/1 -> v_hat/1
  Math Function/1 -> Product/2
  "v  "/1 -> Dot Product/2, Dot Product/1, Product/1
  Switch/1 -> Math Function/1
  sqrt/1 -> Switch/2, Switch/1
  Constant/1 -> Switch/3

== system aausat3_lib/On-board Software/Orbit and Magnetic field models/(IGRF) Magnetic field/Magnetic field model ==
  R_sc(E) : Inport
  S-Function : S-Function  FunctionName=igrfS  Parameters=(((init_jd)/365.25)-4712),igrf_order  EnableBusSupport=off
  B(E) : Outport
  wires:
  R_sc(E)/1 -> S-Function/1
  S-Function/1 -> B(E)/1

== system aausat3_lib/On-board Software/Orbit and Magnetic field models/(IGRF) Magnetic field/Vector rotation by q ==
  q : Inport
  V : Inport  Port=2
  Constant : Constant  Value=0
  Demux : Demux  Outputs=3
  Demux1 : Demux
  Mux : Mux
  Mux1 : Mux  Inputs=3
  Quaternion inverter : Subsystem
  Quaternion mulitiplication : S-Function  FunctionName=qmul  EnableBusSupport=off
  Quaternion mulitiplication1 : S-Function  FunctionName=qmul  EnableBusSupport=off
  Terminator : Terminator
  q'Vq : Outport
  wires:
  Mux1/1 -> q'Vq/1
  Demux1/4 -> Terminator/1
  Demux1/3 -> Mux1/3
  Demux1/2 -> Mux1/2
  Demux1/1 -> Mux1/1
  Quaternion mulitiplication1/1 -> Demux1/1
  Quaternion mulitiplication/1 -> Quaternion mulitiplication1/1
  Mux/1 -> Quaternion mulitiplication/2
  Constant/1 -> Mux/4
  Demux/3 -> Mux/3
  Demux/2 -> Mux/2
  Demux/1 -> Mux/1
  V/1 -> Demux/1
  Quaternion inverter/1(q^-1) -> Quaternion mulitiplication/1
  q/1 -> Quaternion mulitiplication1/2, Quaternion inverter/1(q)

== system aausat3_lib/On-board Software/Orbit and Magnetic field models/Eclipse model/To unit vector ==
  "v  " : Inport
  Constant : Constant
  Dot Product : DotProduct  InputSameDT=on  OutDataTypeStr=Inherit: Inherit via internal rule
  Math Function : Math  Operator=reciprocal  SaturateOnIntegerOverflow=on
  Product : Product  SaturateOnIntegerOverflow=on  OutDataTypeStr=Inherit: Same as first input
  Switch : Switch  Criteria=u2 ~= 0  SaturateOnIntegerOverflow=on
  sqrt : Math  Operator=sqrt  SaturateOnIntegerOverflow=on
  v_hat : Outport
  wires:
  Dot Product/1 -> sqrt/1
  Product/1 -> v_hat/1
  Math Function/1 -> Product/2
  "v  "/1 -> Dot Product/2, Dot Product/1, Product/1
  Switch/1 -> Math Function/1
  sqrt/1 -> Switch/2, Switch/1
  Constant/1 -> Switch/3

== system aausat3_lib/On-board Software/Orbit and Magnetic field models/Eclipse model/To unit vector1 ==
  "v  " : Inport
  Constant : Constant
  Dot Product : DotProduct  InputSameDT=on  OutDataTypeStr=Inherit: Inherit via internal rule
  Math Function : Math  Operator=reciprocal  SaturateOnIntegerOverflow=on
  Product : Product  SaturateOnIntegerOverflow=on  OutDataTypeStr=Inherit: Same as first input
  Switch : Switch  Criteria=u2 ~= 0  SaturateOnIntegerOverflow=on
  sqrt : Math  Operator=sqrt  SaturateOnIntegerOverflow=on
  v_hat : Outport
  wires:
  Dot Product/1 -> sqrt/1
  Product/1 -> v_hat/1
  Math Function/1 -> Product/2
  "v  "/1 -> Dot Product/2, Dot Product/1, Product/1
  Switch/1 -> Math Function/1
  sqrt/1 -> Switch/2, Switch/1
  Constant/1 -> Switch/3

== system aausat3_lib/On-board Software/Orbit and Magnetic field models/SGP4 position/TLE -> JD converter ==
  TLE (Epoch time) : Inport
  Add century : Constant  Value=1900
  Add century1 : Constant  Value=2000
  Gain1 : Gain  Gain=1/1000
  Gain2 : Gain  Gain=1/1000
  Gain3 : Gain  Gain=1000
  Sum1 : Sum  Inputs=++|
  Sum3 : Sum  Inputs=++|
  Sum4 : Sum  Inputs=++-
  Sum5 : Sum  Inputs=|+-
  calculate JD for given year  at 1. jan time 00.00 : Fcn  Expr=367*u(1)-floor(7*(u(1)+floor((1+9)/12))/4)+floor(275*1/9)+1+1721013.5+0/24
  extract year : Rounding
  substract 1 day : Constant
  year 1950-1999 or  2000-2049? : Switch  Criteria=u2 > Threshold  Threshold=50
  JD : Outport
  wires:
  Add century/1 -> Sum3/1
  Gain2/1 -> Sum3/2, year 1950-1999 or  2000-2049?/2
  TLE (Epoch time)/1 -> Gain2/1, Gain1/1
  extract year/1 -> Sum5/2, calculate JD for given year  at 1. jan time 00.00/1
  calculate JD for given year  at 1. jan time 00.00/1 -> Sum4/2
  Sum5/1 -> Gain3/1
  Sum4/1 -> JD/1
  Gain3/1 -> Sum4/1
  substract 1 day/1 -> Sum4/3
  Add century1/1 -> Sum1/1
  Gain1/1 -> Sum1/2
  year 1950-1999 or  2000-2049?/1 -> extract year/1, Sum5/1
  Sum1/1 -> year 1950-1999 or  2000-2049?/3
  Sum3/1 -> year 1950-1999 or  2000-2049?/1

== system aausat3_lib/On-board Software/Orbit and Magnetic field models/Vector rotation by q/Quaternion inverter ==
  q : Inport
  Demux : Demux
  Demux1 : Demux  Outputs=3
  Gain : Gain  Gain=-1  SaturateOnIntegerOverflow=on  OutDataTypeStr=Inherit: Same as input  ParamDataTypeStr=Inherit: Same as input
  Mux : Mux
  Mux1 : Mux  Inputs=3
  q^-1 : Outport
  wires:
  Gain/1 -> Demux1/1
  Demux1/3 -> Mux/3
  Demux1/2 -> Mux/2
  Demux1/1 -> Mux/1
  Mux1/1 -> Gain/1
  Demux/3 -> Mux1/3
  Demux/2 -> Mux1/2
  Demux/1 -> Mux1/1
  Demux/4 -> Mux/4
  Mux/1 -> q^-1/1
  q/1 -> Demux/1

== system aausat3_lib/Sensor Emulation/Magnetometers/Vector rotation by q/Quaternion inverter ==
  q : Inport
  Demux : Demux
  Demux1 : Demux  Outputs=3
  Gain : Gain  Gain=-1  SaturateOnIntegerOverflow=on  OutDataTypeStr=Inherit: Same as input  ParamDataTypeStr=Inherit: Same as input
  Mux : Mux
  Mux1 : Mux  Inputs=3
  q^-1 : Outport
  wires:
  Gain/1 -> Demux1/1
  Demux1/3 -> Mux/3
  Demux1/2 -> Mux/2
  Demux1/1 -> Mux/1
  Mux1/1 -> Gain/1
  Demux/3 -> Mux1/3
  Demux/2 -> Mux1/2
  Demux/1 -> Mux1/1
  Demux/4 -> Mux/4
  Mux/1 -> q^-1/1
  q/1 -> Demux/1

== system aausat3_lib/Sensor Emulation/Sun sensors/Vector rotation by q/Quaternion inverter ==
  q : Inport
  Demux : Demux
  Demux1 : Demux  Outputs=3
  Gain : Gain  Gain=-1  SaturateOnIntegerOverflow=on  OutDataTypeStr=Inherit: Same as input  ParamDataTypeStr=Inherit: Same as input
  Mux : Mux
  Mux1 : Mux  Inputs=3
  q^-1 : Outport
  wires:
  Gain/1 -> Demux1/1
  Demux1/3 -> Mux/3
  Demux1/2 -> Mux/2
  Demux1/1 -> Mux/1
  Mux1/1 -> Gain/1
  Demux/3 -> Mux1/3
  Demux/2 -> Mux1/2
  Demux/1 -> Mux1/1
  Demux/4 -> Mux/4
  Mux/1 -> q^-1/1
  q/1 -> Demux/1

== system aausat3_lib/Disturbances/Atmospheric/Density7/Unit Vector/Vector Mag ==
  Vector : Inport
  Demux : Demux  Outputs=3
  Math Function : Math  Operator=magnitude^2  SaturateOnIntegerOverflow=on
  Math Function1 : Math  Operator=sqrt  SaturateOnIntegerOverflow=on
  Sum : Sum  Inputs=+++
  Magnitude : Outport
  wires:
  Vector/1 -> Math Function/1
  Math Function1/1 -> Magnitude/1
  Sum/1 -> Math Function1/1
  Demux/3 -> Sum/3
  Demux/2 -> Sum/2
  Demux/1 -> Sum/1
  Math Function/1 -> Demux/1

== system aausat3_lib/On-board Software/Orbit and Magnetic field models/(IGRF) Magnetic field/Vector rotation by q/Quaternion inverter ==
  q : Inport
  Demux : Demux
  Demux1 : Demux  Outputs=3
  Gain : Gain  Gain=-1  SaturateOnIntegerOverflow=on  OutDataTypeStr=Inherit: Same as input  ParamDataTypeStr=Inherit: Same as input
  Mux : Mux
  Mux1 : Mux  Inputs=3
  q^-1 : Outport
  wires:
  Gain/1 -> Demux1/1
  Demux1/3 -> Mux/3
  Demux1/2 -> Mux/2
  Demux1/1 -> Mux/1
  Mux1/1 -> Gain/1
  Demux/3 -> Mux1/3
  Demux/2 -> Mux1/2
  Demux/1 -> Mux1/1
  Demux/4 -> Mux/4
  Mux/1 -> q^-1/1
  q/1 -> Demux/1

== matlab function Orbit and Ephemeris/Ephemeris/Sun Position/MATLAB Function ==
  data: u input double; y output double
function y = fcn(u)
%#codegen

y = sun(u);

== matlab function Math Utilities/Quaternion operations/Rotation from q1 to q2/MATLAB Function ==
  data: u input double; y output double
function y = fcn(u)
%#codegen

y = quatmultiply([u(4) u(1) u(2) u(3)], [u(8) u(5) u(6) u(7)]);

== matlab function Orbit and Ephemeris/ECI->ECEF quaternion/MATLAB Function ==
  data: u input double; y output double
function y = fcn(u)
%#codegen

y = eci2ecef(u);

== matlab function Orbit and Ephemeris/Ephemeris/Moon Position/MATLAB Function ==
  data: u input double; y output double
function y = fcn(u)
%#codegen

y = moon(u);

== matlab function Disturbances/Gravity Gradient Torque/MATLAB Function6 ==
  data: u input double; y output double
function y = fcn(u)
%#codegen

y = norm(u);

== matlab function Disturbances/Gravity Moon/MATLAB Function6 ==
  data: u input double; y output double
function y = fcn(u)
%#codegen

y = norm(u);

== matlab function Disturbances/Gravity Sun/MATLAB Function6 ==
  data: u input double; y output double
function y = fcn(u)
%#codegen

y = norm(u);

== matlab function Disturbances/Atmospheric/MATLAB Function ==
  data: input input double; out output double
function out = atm_drag(input)
%#codegen

    rho = input(1);
    Cd = input(2);
    mass_center = input(3:5);
    v = input(6:8);
    r = input(9:11);
    q1 = input(12);
    q2 = input(13);
    q3 = input(14);
    q4 = input(15);
    
    w = [0 0 0.7292e-4]';
    cv = -cross(w, r);
    
    v = v+cv;
    
    v_u = v/norm(v);

    R_ib = [q1^2-q2^2-q3^2+q4^2, 2*(q1*q2+q3*q4), 2*(q1*q3-q2*q4);
            2*(q1*q2-q3*q4), -q1^2+q2^2-q3^2+q4^2, 2*(q2*q3+q1*q4);
            2*(q1*q3+q2*q4), 2*(q2*q3-q1*q4), -q1^2-q2^2+q3^2+q4^2];
                
    small_plate = [0.0 -0.05 -0.05;
                   0.0  0.05 -0.05;
                   0.0  0.05  0.05;
                   0.0 -0.05  0.05]';

    large_plate = [0.1035 0.0 -0.05;
                  -0.1035 0.0 -0.05;
                  -0.1035 0.0  0.05;
                   0.1035 0.0  0.05]';

    antenna = [0.0    0.005 0.0;
               0.0   -0.005 0.0;
               -0.15 -0.005 0.0;
               -0.15  0.005 0.0]';

    plate_front    = translate(rotate(small_plate, [  0   0   0]), [ 0.1035 0 0]);
    plate_back     = translate(rotate(small_plate, [  0 180   0]), [-0.1035 0 0]);
    plate_left     = translate(rotate(large_plate, [  0   0 180]), [0 -0.05 0]);
    plate_right    = translate(rotate(large_plate, [  0   0   0]), [0  0.05 0]);
    plate_top      = translate(rotate(large_plate, [ 90   0   0]), [0  0 -0.05]);
    plate_bottom   = translate(rotate(large_plate, [-90   0   0]), [0  0  0.05]);
    antenna_top_f    = translate(rotate(antenna, [  0 -45 0]),  [-0.1035  0     0.05]);
    antenna_bottom_f = translate(rotate(antenna, [180  45 0]),  [-0.1035  0    -0.05]);
    antenna_left_f   = translate(rotate(antenna, [-90  0 -45]), [-0.1035 -0.05  0]);
    antenna_right_f  = translate(rotate(antenna, [ 90  0  45]), [-0.1035  0.05  0]);
    antenna_top_b    = translate(rotate(antenna, [180 -45 0]),  [-0.1035  0     0.05]);
    antenna_bottom_b = translate(rotate(antenna, [  0  45 0]),  [-0.1035  0    -0.05]);
    antenna_left_b   = translate(rotate(antenna, [ 90  0 -45]), [-0.1035 -0.05  0]);
    antenna_right_b  = translate(rotate(antenna, [-90  0  45]), [-0.1035  0.05  0]);


    satellite_b = repmat(struct('pol', zeros(3,4)), 14);
    satellite_bc = repmat(struct('pol', zeros(3,4)), 14);
    
    satellite_b(1).pol = plate_front;
    satellite_b(2).pol = plate_back;
    satellite_b(3).pol = plate_left;
    satellite_b(4).pol = plate_right;
    satellite_b(5).pol = plate_top;
    satellite_b(6).pol = plate_bottom;
    satellite_b(7).pol = antenna_top_f;
    satellite_b(8).pol = antenna_top_b;
    satellite_b(9).pol = antenna_bottom_f;
    satellite_b(10).pol = antenna_bottom_b;
    satellite_b(11).pol = antenna_left_f;
    satellite_b(12).pol = antenna_left_b;
    satellite_b(13).pol = antenna_right_f;
    satellite_b(14).pol = antenna_right_b;

    j = 0;
    for i = 1:length(satellite_b)
        ret = polygon_backface_check(satellite_b(i).pol, -R_ib*v_u);
        if sum(sum(ret)) ~= 0
            j = j+1;
            satellite_bc(j).pol = ret;
        end
    end
    
    F = [0 0 0]';
    T = [0 0 0]';
    for i = 1:j
        c = polygon3_centroid(satellite_bc(i).pol)-mass_center;
        A = polygon3_area(satellite_bc(i).pol, R_ib*v_u);
        Ft = -v_u*(rho*Cd*A*norm(v)^2)/2;
        Tt = cross(c, R_ib*Ft);

        F = F + Ft;
        T = T + Tt;
    end
    
    out = [T; F];
    
end

== matlab function Disturbances/Atmospheric/Density7/Embedded MATLAB Function ==
  data: cosn_si2 input double; r input double; rho output double; h output double
function [rho,h] = Density(cosn_si2,r)

ellipsoid = [6378.137e3, 0.081819190842];
x = r(1);
y = r(2);
z = r(3);

Csi=cosn_si2; %Cosn(si/2)
%************************************************************
%Formula taken from ecef2geodetic function of Matlab
% Ellipsoid constants
a  = ellipsoid(1);       % Semimajor axis
e2 = ellipsoid(2) ^ 2;   % Square of first eccentricity
ep2 = e2 / (1 - e2);     % Square of second eccentricity
f = 1 - sqrt(1 - e2);    % Flattening
b = a * (1 - f);         % Semiminor axis

% Longitude
lambda = atan2(y,x);

% Distance from Z-axis
rho = hypot(x,y);

% Bowring's formula for initial parametric (beta) and geodetic (phi) latitudes
beta = atan2(z, (1 - f) * rho);
phi = atan2(z   + b * ep2 * sin(beta).^3,...
            rho - a * e2  * cos(beta).^3);

% Fixed-point iteration with Bowring's formula
% (typically converges within two or three iterations)
betaNew = atan2((1 - f)*sin(phi), cos(phi));
count = 0;
while any(beta(:) ~= betaNew(:)) && count < 5
    beta = betaNew;
    phi = atan2(z   + b * ep2 * sin(beta).^3,...
                rho - a * e2  * cos(beta).^3);
    betaNew = atan2((1 - f)*sin(phi), cos(phi));
    count = count + 1;
end

% Calculate ellipsoidal height from the final value for latitude
sinphi = sin(phi);
N = a ./ sqrt(1 - e2 * sinphi.^2);
h = rho .* cos(phi) + (z + e2 * N .* sinphi) .* sinphi - N;
%*************************************************************************
h=h/1000;%in Km

%% Harris-Priester Density Table
% h(km), rho-min(g/km3), rho-max(g/km3))
HP = [100, 497400, 497400; ...
    120, 24900, 24900; ...
    130, 8377, 8710; ...
    140, 3899, 4059; ...
    150, 2122, 2215; ...
    160, 1263, 1344; ...
    170, 800.80, 875.80; ...
    180, 528.30, 601; ...
    190, 361.70, 429.70; ...
    200, 255.70, 316.20; ...
    210, 183.90, 239.60; ...
    220, 134.10, 185.30; ...
    230, 99.490, 145.50; ...
    240, 74.880, 115.70; ...
    250, 57.090, 93.080; ...
    260, 44.030, 75.550; ...
    270, 34.300, 61.820; ...
    280, 26.970, 50.950; ...
    290, 21.390, 42.260; ...
    300, 17.080, 35.260; ...
    320, 10.990, 25.110; ...
    340, 7.2140, 18.190; ...
    360, 4.8240, 13.370; ...
    380, 3.2740, 9.9550; ...
    400, 2.2490, 7.4920; ...
    420, 1.5580, 5.6840; ...
    440, 1.0910, 4.3550; ...
    460, 0.77010, 3.3620; ...
    480, 0.54740, 2.6120; ...
    500, 0.39160, 2.0420; ...
    520, 0.28190, 1.6050; ...
    540, 0.20420, 1.2670; ...
    560, 0.14880, 1.0050; ...
    580, 0.10920, 0.79970; ...
    600, 0.080700, 0.63900; ...
    620, 0.060120, 0.51230; ...
    640, 0.045190, 0.41210; ...
    660, 0.034300, 0.33250; ...
    680, 0.026320, 0.26910; ...
    700, 0.020430, 0.21850; ...
    720, 0.016070, 0.17790; ...
    740, 0.012810, 0.14520; ...
    760, 0.010360, 0.11900; ...
    780, 0.0084960, 0.097760; ...
    800, 0.0070690, 0.080590; ...
    840, 0.0046800, 0.057410; ...
    880, 0.0032000, 0.042100; ...
    920, 0.0022100, 0.031300; ...
    960, 0.0015600, 0.023600; ...
    1000, 0.0011500, 0.018100];
%%
if h>HP(end,1)
    error('Too high altitude');
    rho=0;
elseif h<HP(1,1)
    error('Too low altitude');
    rho=0;
else
    indxi=find(HP(:,1)<=h);
    hi=HP(indxi(end),1);
    rho_m_i=HP(indxi(end),2);
    rho_M_i=HP(indxi(end),3);
    
    indxii=find(HP(:,1)>=h);
    hii=HP(indxii(1),1);
    rho_m_ii=HP(indxii(1),2);
    rho_M_ii=HP(indxii(1),3);
    
    Hm=(hi-hii)/log(rho_m_ii/rho_m_i);
    HM=(hi-hii)/log(rho_M_ii/rho_M_i);
    
    rho_m=rho_m_i*exp((hi-h)/Hm);
    rho_M=rho_M_i*exp((hi-h)/HM);
    
    rho=rho_m+((rho_M-rho_m)*Csi);
    rho=rho/1e12; %in Kg/m3
end

== matlab function Disturbances/Atmospheric/Density7/Subsystem/R.Ascen & Declination in rads ==
  data: jd input double; rtasc output double; decl output double
function [rtasc,decl] = sun ( jd )

        twopi      =     2.0*pi;
        deg2rad    =     pi/180.0;

        % -------------------------  implementation   -----------------
        % -------------------  initialize values   --------------------
        tut1= ( jd - 2451545.0  )/ 36525.0;
%fprintf(1,'tut1 %14.9f \n',tut1);

        meanlong= 280.460  + 36000.77*tut1;
        meanlong= rem( meanlong,360.0  );  %deg

        ttdb= tut1;
        meananomaly= 357.5277233  + 35999.05034 *ttdb;
        meananomaly= rem( meananomaly*deg2rad,twopi );  %rad
        if ( meananomaly < 0.0  )
            meananomaly= twopi + meananomaly;
          end

        eclplong= meanlong + 1.914666471 *sin(meananomaly) ...
                    + 0.019994643 *sin(2.0 *meananomaly); %deg

        obliquity= 23.439291  - 0.0130042 *ttdb;  %deg

        meanlong = meanlong*deg2rad;
        if ( meanlong < 0.0  )
            meanlong= twopi + meanlong;
          end
        eclplong = eclplong *deg2rad;
        obliquity= obliquity *deg2rad;

        % --------- find magnitude of sun vector, )   components ------
        magr= 1.000140612  - 0.016708617 *cos( meananomaly ) ...
                              - 0.000139589 *cos( 2.0 *meananomaly );    % in au's

%         rsun(1)= magr*cos( eclplong );
%         rsun(2)= magr*cos(obliquity)*sin(eclplong);
%         rsun(3)= magr*sin(obliquity)*sin(eclplong);

%fprintf(1,'meanlon %11.6f meanan %11.6f eclplon %11.6f obli %11.6f \n', ...
           %meanlong/deg2rad,meananomaly/deg2rad,(2.0*pi+eclplong)/deg2rad,obliquity/deg2rad);
%fprintf(1,'rs %11.9f %11.9f %11.9f \n',rsun);
%fprintf(1,'magr %14.7f \n',magr);
%%%%rsun
%%%%rsun*149597870.0

        rtasc= atan( cos(obliquity)*tan(eclplong) );

        % --- check that rtasc is in the same quadrant as eclplong ----
        if ( eclplong < 0.0  )
            eclplong= eclplong + twopi;    % make sure it's in 0 to 2pi range
          end
        if ( abs( eclplong-rtasc ) > pi*0.5  )
            rtasc= rtasc + 0.5 *pi*round( (eclplong-rtasc)/(0.5 *pi));
          end
%fprintf(1,'rtasc %11.6f \n',rtasc/deg2rad);
        decl = asin( sin(obliquity)*sin(eclplong) );
%fprintf(1,'decl %11.6f \n',decl/deg2rad);

== matlab function AAUSAT3/inc from TLE ==
  data: u input double; y output double
function y = fcn(u)
%#codegen

y = u(7);
